simulink model "ep_5_2"  (R2023b)
settings: Solver=VariableStepAuto  StartTime=0.0  StopTime=10.0  MaxStep=0.01  RelTol=1e-3
settings Model: Creator=86186  LastModifiedBy=86186

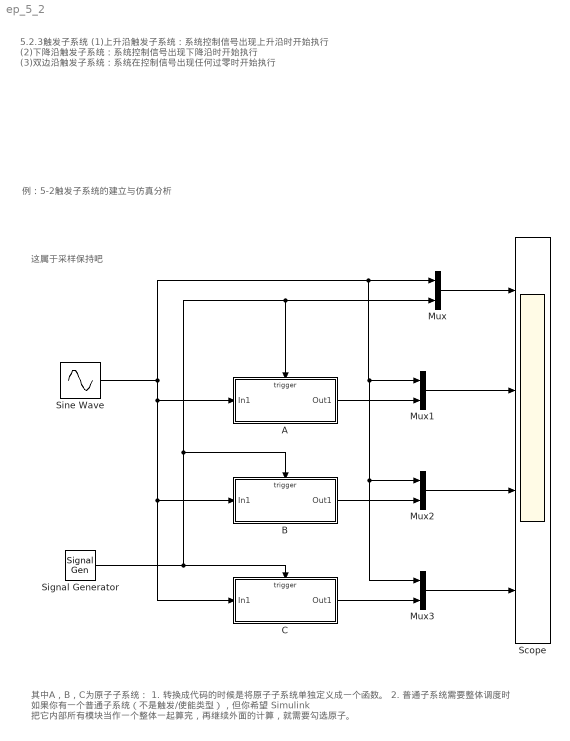
== system ep_5_2 ==
  note: 其中A，B，C为原子子系统：
      | 1. 转换成代码的时候是将原子子系统单独定义成一个函数。
      | 2. 普通子系统需要整体调度时
      | 如果你有一个普通子系统（不是触发/使能类型），但你希望 Simulink 把它内部所有模块当作一个整体一起算完，再继续外面的计算，就需要勾选原子。
  note: 这属于采样保持吧
  note: 例：5-2触发子系统的建立与仿真分析
  note: 5.2.3触发子系统
      | (1)上升沿触发子系统：系统控制信号出现上升沿时开始执行
      | (2)下降沿触发子系统：系统控制信号出现下降沿时开始执行
      | (3)双边沿触发子系统：系统在控制信号出现任何过零时开始执行
  A : Subsystem  TreatAsAtomicUnit=on
  B : Subsystem  TreatAsAtomicUnit=on
  C : Subsystem  TreatAsAtomicUnit=on
  Mux{,1..3} (4 alike) : Mux  Inputs=2
  Scope : Scope  NumInputPorts=4
  Signal Generator : SignalGenerator  WaveForm=square
  Sine Wave : Sin  Frequency=8  SampleTime=0
  wires:
  Signal Generator/1 -> C/Trigger, B/Trigger, A/Trigger, Mux/2
  Mux/1 -> Scope/1
  Sine Wave/1 -> C/1(In1), B/1(In1), A/1(In1), Mux3/1, Mux2/1, Mux1/1, Mux/1
  C/1(Out1) -> Mux3/2
  Mux3/1 -> Scope/4
  B/1(Out1) -> Mux2/2
  A/1(Out1) -> Mux1/2
  Mux1/1 -> Scope/2
  Mux2/1 -> Scope/3

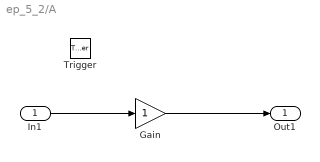
== system ep_5_2/A ==
  In1 : Inport
  Trigger : TriggerPort  VariantControl=(inherit)
  Gain : Gain
  Out1 : Outport
  wires:
  In1/1 -> Gain/1
  Gain/1 -> Out1/1

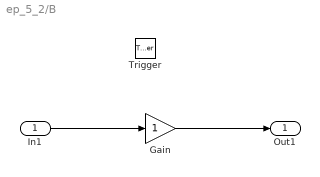
== system ep_5_2/B ==
  In1 : Inport
  Trigger : TriggerPort  TriggerType=falling  VariantControl=(inherit)
  Gain : Gain
  Out1 : Outport
  wires:
  In1/1 -> Gain/1
  Gain/1 -> Out1/1

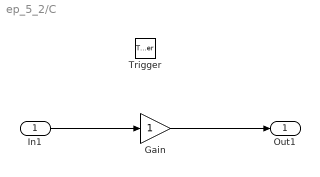
== system ep_5_2/C ==
  In1 : Inport
  Trigger : TriggerPort  TriggerType=either  VariantControl=(inherit)
  Gain : Gain
  Out1 : Outport
  wires:
  In1/1 -> Gain/1
  Gain/1 -> Out1/1
